simulink model "plant_harness"  (R2019b)
settings: Solver=VariableStepAuto  StartTime=0.0  StopTime=50  RelTol=1e-3
undefined symbols (not defined in the file): sigbuilder_block
settings Model: Creator=nmb  LastModifiedBy=nmb

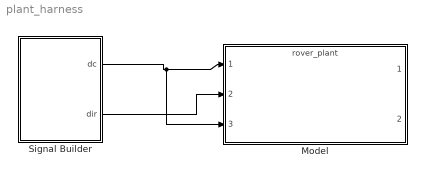
== system plant_harness ==
  Model : ModelReference  ModelNameDialog=rover_plant  SimulationMode=Normal  ModelReferenceVersion=1.9
  Signal Builder : Subsystem  Tag=STV Subsys  LoadFcn=sigbuilder_block('load',[437.6 199.2 550.4 400 ]);  StartFcn=sigbuilder_block('start');  StopFcn=sigbuilder_block('stop');  ClipboardFcn=sigbuilder_block('clipboard');  mask(Sigbuilder block){tuvar=[0:10]}
      mask help: Simulink:masks:SigbuilderBlock_MD
      mask init:
      | if ~strcmp(get_param(bdroot(gcbh),'SimulationStatus'),'stopped') tuvar = sigbuilder_block('maskInit'); end
      settings: CopyFcn=sigbuilder_block('copy');  DeleteFcn=sigbuilder_block('delete');  ModelCloseFcn=sigbuilder_block('modelClose');  PreSaveFcn=sigbuilder_block('preSave');  PauseFcn=sigbuilder_block('pause');  ContinueFcn=sigbuilder_block('continue');  NameChangeFcn=sigbuilder_block('namechange');  OpenFcn=sigbuilder_block('open',[437.6 199.2 550.4 400 ]);  CloseFcn=sigbuilder_block('close');
      mask Display: plot(0, 0, 100, 100,[2, 2, 32, 32, 2], [68, 8, 8, 68, 68],[32, 2], [38, 38], [32, 19, 2],[53, 60, 44], [32, 17, 17, 2],[16, 16, 31, 31]);txt = getActiveGroup(gcbh);text(2, 100, txt,'verticalAlignment', 'top');
  wires:
  Signal Builder/1(dc) -> Model/3, Model/1
  Signal Builder/2(dir) -> Model/2

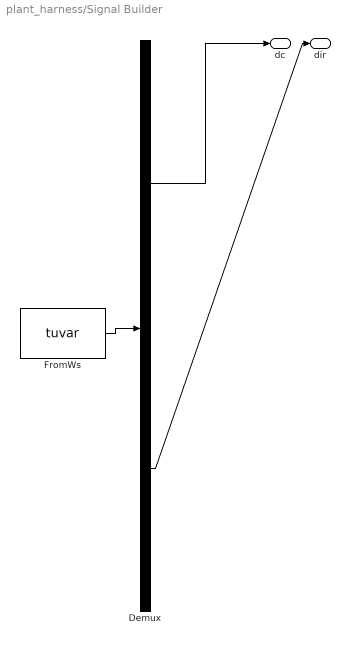
== system plant_harness/Signal Builder ==
  Demux : Demux  Tag=STV Demux  Outputs=2
  FromWs : FromWorkspace  Tag=STV FromWs  VariableName=tuvar  SampleTime=0
      SigBuilderData=|
      | common.afterFinalStr = 'Extrapolate'
      | common.sampleTime = 0
      | dataSet.timeRange = [0 50]
      | dataSet.name = 'Group 1'
      | sbobj.Groups.Name = 'Group 1'
      | sbobj.Groups.Signals(1).Name = 'dc'
      | sbobj.Groups.Signals(1).XData = [0 7 12 12 21.6 25.2 27.5 34.2 38.5 41.5 41.5 47.9 50]
      | sbobj.Groups.Signals(1).YData = [0 1 1 0 0 0.45 0 0 0.88 0.88 0.87 0 0]
      | sbobj.Groups.Signals(2).Name = 'dir'
      | sbobj.Groups.Signals(2).XData = [0 1.2 1.2 17.8 17.8 31.3 31.3 45.6 45.6 50]
      | sbobj.Groups.Signals(2).YData = [0 0 1 1 0.02 0.02 -1 -1 0 0]
      | sbobj.Groups.TimeRange = [0 50]
  dc : Outport  Tag=STV Outport
  dir : Outport  Tag=STV Outport  Port=2
  wires:
  Demux/1 -> dc/1
  FromWs/1 -> Demux/1
  Demux/2 -> dir/1
